simulink model "quant_model"  (R2014a)
settings: Solver=ode45  StartTime=0.0  StopTime=30.0  RelTol=1e-3
values from neighbouring files (symbols this model uses):
  d = str2num(get(handles.ds_tag, 'String'))    [enter_paprameters.m]    (also in input_tf2.m = str2num(ds); quantization.m; test.m = [1 1])
  d_d = [1 1]    [test.m]
  n = str2num(get(handles.ns_tag, 'String'))    [enter_paprameters.m]    (also in input_tf2.m = str2num(ns); quantization.m; test.m = [1])
  n_d = [1]    [test.m]
  u_d = 1    [main.m]    (also in test.m)
undefined symbols (not defined in the file or in its folder): cd, cn
settings Model: Creator=Alexey  LastModifiedBy=Alexey
settings SolverCC: ZeroCrossControl=EnableAll

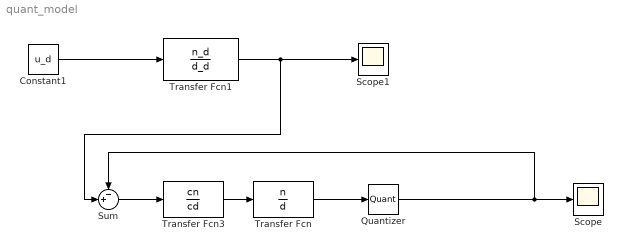
== system quant_model ==
  Constant1 : Constant  Value=u_d
  Quantizer : Quantizer  QuantizationInterval=delta
  Scope : Scope
      settings: SaveName=out
  Scope1 : Scope
      settings: SaveName=out_d
  Sum : Sum  Inputs=-+|
  Transfer Fcn : TransferFcn  Numerator=n  Denominator=d
  Transfer Fcn1 : TransferFcn  Numerator=n_d  Denominator=d_d
  Transfer Fcn3 : TransferFcn  Numerator=cn  Denominator=cd
  wires:
  Transfer Fcn/1 -> Quantizer/1
  Constant1/1 -> Transfer Fcn1/1
  Transfer Fcn1/1 -> Sum/2, Scope1/1
  Sum/1 -> Transfer Fcn3/1
  Transfer Fcn3/1 -> Transfer Fcn/1
  Quantizer/1 -> Sum/1, Scope/1
